simulink model "Ex4"  (R2022b)
settings: Solver=VariableStepAuto  StartTime=0.0  StopTime=10.0  RelTol=1e-3
settings Model: Creator=felix  LastModifiedBy=felix

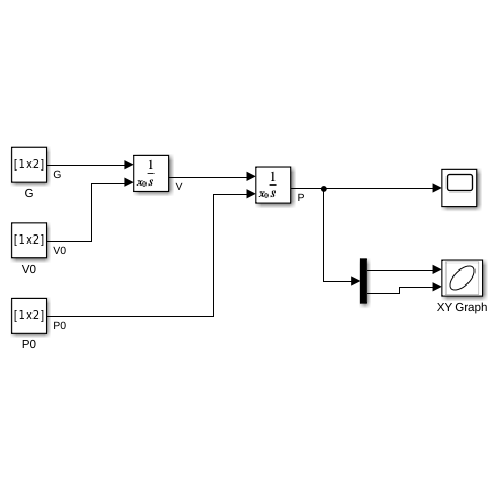
[thumbnail: Simulink's stored preview of the top-level diagram]
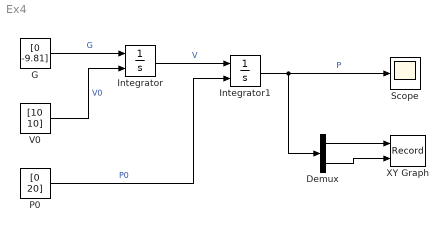
== system Ex4 ==
  Demux : Demux  Outputs=2
  G : Constant  Value=[0 -9.81]
  Integrator : Integrator  InitialConditionSource=external
  Integrator1 : Integrator  InitialConditionSource=external
  P0 : Constant  Value=[0 20]
  Scope : Scope
  V0 : Constant  Value=[10 10]
  XY Graph : Record  FileSettingsInternal="{\"entries\":[{\"content\":{\"excelSettings\":{\"content\":{},\"type\":\"Streamout.ExcelSettings\"}},\"type\":\"Streamout.FileSettingStorage\",\"uuid\":\"b43cbfd5-361a-4a01-b94e-05a5c7c4d5aa\"}],\"packageUris\":[\"http://schema.mathworks.com/mf0/streamout_blocks/R2020a\"],\"version\":\"1.0\"}"  Layout=[1 1]  SignalsInternal="{\"entries\":[{\"content\":{\"signals\":[{\"content\":{\"blockPath\":[\"untitled/XY Graph\"],\"channel\":[],\"dimensions\":[1],\"domain\":\"untitled/XY Graph\",\"lineColor\":\"#a2142f\",\"plots\":[1],\"port\":1,\"sid\":[\"\"],\"signalID\":31,\"signalName\":\"Demux:1\"},\"type\":\"RecordBlkView.Signal\",\"uuid\":\"7e464f07-3493-47e3-a3ac-9783e36463a8\"},{\"content\":{\"blockPath\":[\"untitled/XY Graph\"],\"channel\":[],\"dimensions\":[1],\"domain\":\"untitled/XY Graph\",\"lineColor\":\"#139fff\",\"plots\":[1],\"port\":2,\"sid\":[\"\"],\"signalID\":35,\"signalName\":\"Demux:2\"},\"type\":\"RecordBlkView.Signal\",\"uuid\":\"a7c96423-a875-41ea-bc65-1457a2fd38f6\"}]},\"type\":\"RecordBlkView.InputSignals\",\"uuid\":\"1aa01b1b-4796-4180-9c72-c851bbf67158\"}],\"packageUris\":[\"http://schema.mathworks.com/mf0/streamout_blocks/R2020a\"],\"version\":\"1.0\"}"  VisualizationBindings="{\"xyplotplugin\":{\"info\":[{\"series\":[{\"bindingParametersList\":[{\"parameter\":\"X-Axis\",\"signalID\":31,\"signalName\":\"Demux:1\"},{\"parameter\":\"Y-Axis\",\"signalID\":35,\"signalName\":\"Demux:2\"}],\"seriesID\":45096}],\"subplotID\":1}]}}"  CompatibilityTag=XY
  wires:
  G/1 -> Integrator/1  "G"
  Integrator/1 -> Integrator1/1  "V"
  V0/1 -> Integrator/2  "V0"
  P0/1 -> Integrator1/2  "P0"
  Integrator1/1 -> Demux/1, Scope/1  "P"
  Demux/1 -> XY Graph/1
  Demux/2 -> XY Graph/2
